simulink library "SixDoFDynamicsQuat_cl"  (R2020a)
settings: Solver=VariableStepAuto  StartTime=0.0  StopTime=10.0  RelTol=1e-3
undefined symbols (not defined in the file): initAngRates, Veh
libraries: vrlib x2, eulAng2RotMat_ul x1, vectorNormalizer_ul x1, quat2RotMat_ul x1, quat2EulerAng_ul x1, rotMat2Quat_ul x1
settings Model: Creator=mcobb  LastModifiedBy=John Jr
settings DataIOCC: ReturnWorkspaceOutputs=off
settings DebuggingCC: ArithmeticOperatorsInVariantConditions=warning
settings SFSimCC: CustomCodeUndefinedFunction=UseInterfaceOnly

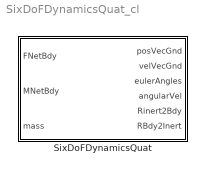
== system SixDoFDynamicsQuat_cl ==
  SixDoFDynamicsQuat : Subsystem  mask{J=Veh.inertia_CM.Value, initPos=Veh.initPosVecGnd.Value, initVel=Veh.initVelVecBdy.Value, initEulAngs=Veh.initEulAng.Value, initAngVel=Veh.initAngVelVec.Value}
      mask prompts: J "Inertia matrix"; initPos "Initial position"; initVel "Initial velocity"; initEulAngs "Initial Euler Angles"; initAngVel "Initial Angular Velocity Vec"
      mask init:
      | Jinv = inv(J);

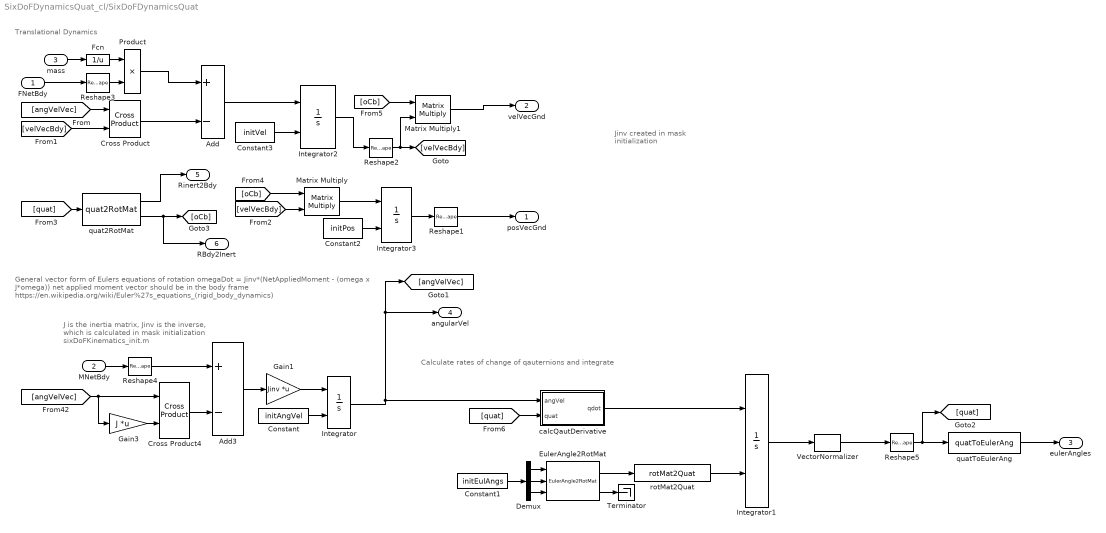
== system SixDoFDynamicsQuat_cl/SixDoFDynamicsQuat ==
  note: Translational Dynamics
  note: Calculate rates of change of qauternions and integrate
  note: General vector form of Eulers equations of rotation
      | omegaDot = Jinv*(NetAppliedMoment - (omega x J*omega))
      | net applied moment vector should be in the body frame
      | https://en.wikipedia.org/wiki/Euler%27s_equations_(rigid_body_dynamics)
  note: J is the inertia matrix, Jinv is the inverse,
      | which is calculated in mask initialization
      | sixDoFKinematics_init.m
  note: Jinv created in mask initialization
  FNetBdy : Inport
  MNetBdy : Inport  Port=2
  mass : Inport  Port=3
  Add : Sum  Inputs=+-
  Add3 : Sum  Inputs=+-
  Constant : Constant  Value=initAngVel
  Constant1 : Constant  Value=initEulAngs
  Constant2 : Constant  Value=initPos
  Constant3 : Constant  Value=initVel
  Cross Product : vrlib/Utilities/Cross Product
  Cross Product4 : vrlib/Utilities/Cross Product
  Demux : Demux  Outputs=3
  EulerAngle2RotMat : eulAng2RotMat_ul/EulerAngle2RotMat  SystemSampleTime=-1  Latency=0  AutoFrameSizeCalculation=off
  Fcn : Fcn  Expr=1/u
  Gain1 : Gain  Gain=Jinv  Multiplication=Matrix(K*u)
  Gain3 : Gain  Gain=J  Multiplication=Matrix(K*u)
  Integrator : Integrator  InitialConditionSource=external  InitialCondition=initAngRates
  Integrator1 : Integrator  InitialConditionSource=external  InitialCondition=initEulAngs
  Integrator2 : Integrator  InitialConditionSource=external  InitialCondition=initVel
  Integrator3 : Integrator  InitialConditionSource=external  InitialCondition=initPos
  Matrix Multiply : Product  Multiplication=Matrix(*)
  Matrix Multiply1 : Product  Multiplication=Matrix(*)
  Product : Product
  Reshape{1..5} (5 alike) : Reshape  OutputDimensionality=Column vector (2-D)
  Terminator : Terminator
  "VectorNormalizer " : vectorNormalizer_ul/VectorNormalizer   SystemSampleTime=-1  Latency=0  AutoFrameSizeCalculation=off
  calcQautDerivative : Subsystem
  quat2RotMat : quat2RotMat_ul/quat2RotMat  SystemSampleTime=-1  Latency=0  AutoFrameSizeCalculation=off
  quatToEulerAng : quat2EulerAng_ul/quatToEulerAng  SystemSampleTime=-1  Latency=0  AutoFrameSizeCalculation=off
  rotMat2Quat : rotMat2Quat_ul/rotMat2Quat  SystemSampleTime=-1  Latency=0  AutoFrameSizeCalculation=off
  posVecGnd : Outport  VectorParamsAs1DForOutWhenUnconnected=off
  velVecGnd : Outport  Port=2  VectorParamsAs1DForOutWhenUnconnected=off
  eulerAngles : Outport  Port=3  VectorParamsAs1DForOutWhenUnconnected=off
  angularVel : Outport  Port=4  VectorParamsAs1DForOutWhenUnconnected=off
  Rinert2Bdy : Outport  Port=5  VectorParamsAs1DForOutWhenUnconnected=off
  RBdy2Inert : Outport  Port=6  VectorParamsAs1DForOutWhenUnconnected=off
  wires:
  Reshape4/1 -> Add3/1
  [oCb] -> Matrix Multiply1/1
  Reshape1/1 -> posVecGnd/1
  Constant3/1 -> Integrator2/2
  Matrix Multiply1/1 -> velVecGnd/1
  [oCb] -> Matrix Multiply/1
  Cross Product4/1 -> Add3/2
  Integrator1/1 -> "VectorNormalizer "/1
  Integrator/1 -> calcQautDerivative/1(angVel), angularVel/1, [angVelVec]
  MNetBdy/1 -> Reshape4/1
  Cross Product/1 -> Add/2
  Add/1 -> Integrator2/1
  [velVecBdy] -> Cross Product/2
  Matrix Multiply/1 -> Integrator3/1
  Add3/1 -> Gain1/1
  [velVecBdy] -> Matrix Multiply/2
  Reshape5/1 -> quatToEulerAng/1, [quat]
  [angVelVec] -> Cross Product4/1, Gain3/1
  Constant2/1 -> Integrator3/2
  Integrator2/1 -> Reshape2/1
  FNetBdy/1 -> Reshape3/1
  calcQautDerivative/1(qdot) -> Integrator1/1
  [angVelVec] -> Cross Product/1
  Gain3/1 -> Cross Product4/2
  Reshape2/1 -> Matrix Multiply1/2, [velVecBdy]
  Constant/1 -> Integrator/2
  Constant1/1 -> Demux/1
  Gain1/1 -> Integrator/1
  Integrator3/1 -> Reshape1/1
  [quat] -> quat2RotMat/1
  rotMat2Quat/1 -> Integrator1/2
  quatToEulerAng/1 -> eulerAngles/1
  [quat] -> calcQautDerivative/2(quat)
  quat2RotMat/2 -> RBdy2Inert/1, [oCb]
  quat2RotMat/1 -> Rinert2Bdy/1
  Demux/1 -> EulerAngle2RotMat/1
  Demux/2 -> EulerAngle2RotMat/2
  Demux/3 -> EulerAngle2RotMat/3
  EulerAngle2RotMat/1 -> rotMat2Quat/1
  EulerAngle2RotMat/2 -> Terminator/1
  "VectorNormalizer "/1 -> Reshape5/1
  mass/1 -> Fcn/1
  Fcn/1 -> Product/1
  Reshape3/1 -> Product/2
  Product/1 -> Add/1

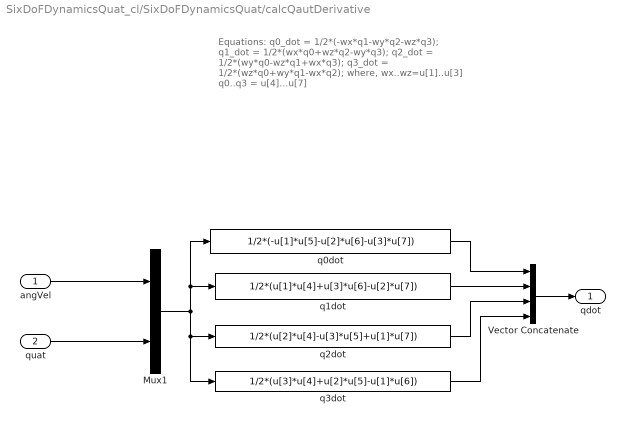
== system SixDoFDynamicsQuat_cl/SixDoFDynamicsQuat/calcQautDerivative ==
  note: Equations:
      | q0_dot = 1/2*(-wx*q1-wy*q2-wz*q3);
      | q1_dot = 1/2*(wx*q0+wz*q2-wy*q3);
      | q2_dot = 1/2*(wy*q0-wz*q1+wx*q3);
      | q3_dot = 1/2*(wz*q0+wy*q1-wx*q2);
      |
      | where,
      | wx..wz=u[1]..u[3]
      | q0..q3 = u[4]...u[7]
  angVel : Inport
  quat : Inport  Port=2
  Mux1 : Mux  Inputs=[3 4]
  Vector Concatenate : Concatenate  NumInputs=4
  q0dot : Fcn  Expr=1/2*(-u[1]*u[5]-u[2]*u[6]-u[3]*u[7])
  q1dot : Fcn  Expr=1/2*(u[1]*u[4]+u[3]*u[6]-u[2]*u[7])
  q2dot : Fcn  Expr=1/2*(u[2]*u[4]-u[3]*u[5]+u[1]*u[7])
  q3dot : Fcn  Expr=1/2*(u[3]*u[4]+u[2]*u[5]-u[1]*u[6])
  qdot : Outport  PortDimensions=[4,1]  VectorParamsAs1DForOutWhenUnconnected=off
  wires:
  quat/1 -> Mux1/2
  q3dot/1 -> Vector Concatenate/4
  Vector Concatenate/1 -> qdot/1
  q2dot/1 -> Vector Concatenate/3
  q1dot/1 -> Vector Concatenate/2
  q0dot/1 -> Vector Concatenate/1
  angVel/1 -> Mux1/1
  Mux1/1 -> q2dot/1, q3dot/1, q0dot/1, q1dot/1
